simulink model "DemoCordic"  (Simulink 6.3)
settings: Solver=FixedStepDiscrete  SolverMode=SingleTasking  StartTime=0.0  StopTime=137*20*8  FixedStep=1  RelTol=1e-3
PreLoadFcn:
  | cordic_precision=20;
  | ScalingFactor = (2^(cordic_precision-1))-1;
  | K=1.0;
  | for i=1:cordic_precision
  |   cordic_atan_table(i) = round(atan(K)*ScalingFactor);
  |   K=0.5*K;
  | end;
  | disp(['cordic_precision =' num2str(cordic_precision)]);
  | disp(['cordic_atan_table =' num2str(cordic_atan_table)]);
InitFcn:
  | %% DSPBuilder Start
  | alt_dspbuilder_update_model(bdroot)
  | %% DSPBuilder End
libraries: allblocks_alteradspbuilder2 x51
settings Model: LastModifiedBy=LKONG  StrictBusMsg=None
settings DataIOCC: SignalLoggingName=sigsOut
settings OptimizationCC: InlineInvariantSignals=on
settings DebuggingCC: SolverPrmCheckMsg=none
settings HardwareCC: TargetUnknown=on

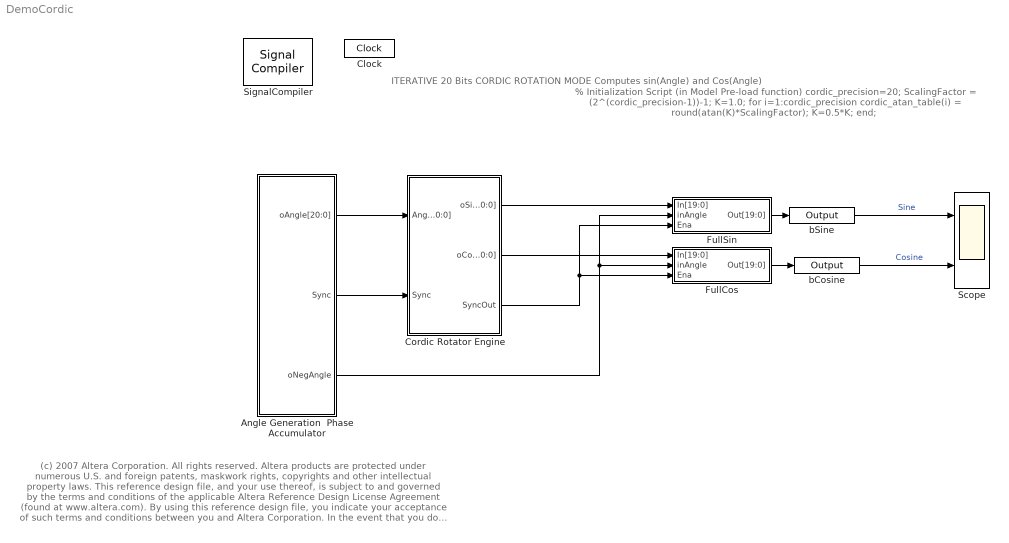
== system DemoCordic ==
  note: ITERATIVE 20 Bits CORDIC
      | ROTATION MODE
      | Computes sin(Angle) and Cos(Angle)
  note: % Initialization Script (in Model Pre-load function)
      | cordic_precision=20;
      | ScalingFactor = (2^(cordic_precision-1))-1;
      | K=1.0;
      | for i=1:cordic_precision
      |   cordic_atan_table(i) = round(atan(K)*ScalingFactor);
      |   K=0.5*K;
      | end;
  note: (c) 2007 Altera Corporation. All rights reserved.  Altera products are protected under numerous U.S. and foreign patents, maskwork rights, copyrights and other intellectual property laws.
      | This reference design file, and your use thereof, is subject to and governed by the terms and conditions of the applicable Altera Reference Design License Agreement (found at www.altera.com).
      | By using this reference design file, you indicate your acceptance of such terms and conditions between you and Altera Corporation.
      | In the event that you do not agree with such terms and conditions, you may not use the reference design file and please promptly destroy any copies you have made.
      | This reference design file being provided on an "as-is" basis and as an accommodation and therefore all warranties, representations or guarantees of any kind (whether express, implied or statutory)
      | including, without limitation, warranties of merchantability, non-infringement, or fitness for a particular purpose, are specifically disclaimed.
      | By making this reference design file available, Altera expressly does not recommend, suggest or require that this reference design file be used in combination with any other product not provided by Altera
  Angle Generation  Phase Accumulator : Subsystem  AncestorBlock=ALTELINK/AltLab/HDL SubSystem
      mask Type: SubSystem AlteraBlockSet
  Clock : allblocks_alteradspbuilder2/Clock  ClockPeriod=100  ClockPeriodUnit=ns  SampleTime=1  SimulationStartCycle=5  PhaseOffset=0  Reset=aclr  ResetType=Active Low  Export=off
  Cordic Rotator Engine : Subsystem  AncestorBlock=ALTELINK/AltLab/HDL SubSystem
      mask Type: SubSystem AlteraBlockSet
  FullCos : Subsystem  AncestorBlock=ALTELINK/AltLab/HDL SubSystem
      mask Type: SubSystem AlteraBlockSet
  FullSin : Subsystem  AncestorBlock=ALTELINK/AltLab/HDL SubSystem
      mask Type: SubSystem AlteraBlockSet
  Scope : Scope  NumInputPorts=2
      settings: YMin=-750000~-750000  YMax=750000~750000  Decimation=20
  SignalCompiler : allblocks_alteradspbuilder2/Signal Compiler  DeviceFamily=Stratix IV  DeviceName=AUTO  EnableSignalTap=off  SignalTapDepth=128  UseBoardBlock=off  StpUseDefaultClock=on  StpClock=Clock
  bCosine : allblocks_alteradspbuilder2/Output  iofile=d:\wsTrunk\workspace\Documentation\DesignExamples\Demos\Transforms\Cordic\tb_DemoCordic\DemoCordic_bCosine.capture  BusType=Signed Integer  bwl=21  bwr=0  PORTTYPE=Output
  bSine : allblocks_alteradspbuilder2/Output  iofile=d:\wsTrunk\workspace\Documentation\DesignExamples\Demos\Transforms\Cordic\tb_DemoCordic\DemoCordic_bSine.capture  BusType=Signed Integer  bwl=21  bwr=0  PORTTYPE=Output
  wires:
  bCosine/1 -> Scope/2  "Cosine"
  Cordic Rotator Engine/3(SyncOut) -> FullSin/3(Ena), FullCos/3(Ena)
  bSine/1 -> Scope/1  "Sine"
  Angle Generation  Phase Accumulator/2(Sync) -> Cordic Rotator Engine/2(Sync)
  Angle Generation  Phase Accumulator/1(oAngle[20:0]) -> Cordic Rotator Engine/1(Angle[20:0])
  Angle Generation  Phase Accumulator/3(oNegAngle) -> FullSin/2(inAngle), FullCos/2(inAngle)
  FullSin/1(Out[19:0]) -> bSine/1
  Cordic Rotator Engine/1(oSin[20:0]) -> FullSin/1(In[19:0])
  FullCos/1(Out[19:0]) -> bCosine/1
  Cordic Rotator Engine/2(oCos[20:0]) -> FullCos/1(In[19:0])

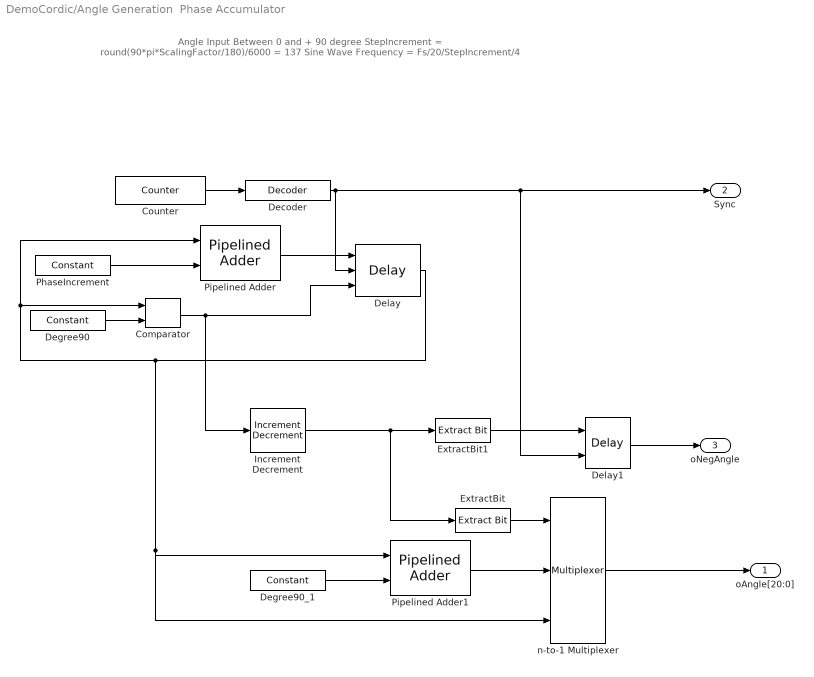
== system DemoCordic/Angle Generation  Phase Accumulator ==
  note: Angle Input Between 0 and + 90 degree
      | StepIncrement = round(90*pi*ScalingFactor/180)/6000 = 137
      | Sine Wave Frequency = Fs/20/StepIncrement/4
  Comparator : allblocks_alteradspbuilder2/Comparator  direction=a > b
  Counter : allblocks_alteradspbuilder2/Counter  BusType=Unsigned Integer  bwl=5  bwr=0  use_modulo=on  modulo=20  SpecifyClock=off  direction=Increment  use_sload=off  use_sset=off  svalue=1  use_clk_ena=off  use_ena=off  use_sclr=off
  Decoder : allblocks_alteradspbuilder2/Decoder  BusType=Unsigned Integer  bwl=5  bwr=0  registered=off  value=0
  Degree90 : allblocks_alteradspbuilder2/Constant  mask_cst=round(90*pi*ScalingFactor/180)  BusType=Signed Integer  bwl=21  bwr=0  SpecifyClock=off
  Degree90_1 : allblocks_alteradspbuilder2/Constant  mask_cst=round(90*pi*ScalingFactor/180)  BusType=Signed Integer  bwl=21  bwr=0  SpecifyClock=off
  Delay : allblocks_alteradspbuilder2/Delay  pipeline=1  ClockPhase=1  use_ena=on  use_sclr=on  use_init=off  reset_value=1
  Delay1 : allblocks_alteradspbuilder2/Delay  pipeline=2  ClockPhase=1  use_ena=on  use_sclr=off  use_init=off  reset_value=1
  ExtractBit : allblocks_alteradspbuilder2/Extract Bit  BusType=Signed Fractional  bwl=2  bwr=0  bitToSelect=0
  ExtractBit1 : allblocks_alteradspbuilder2/Extract Bit  BusType=Signed Fractional  bwl=2  bwr=0  bitToSelect=1
  Increment Decrement : allblocks_alteradspbuilder2/Increment Decrement  BusType=Unsigned Integer  bwl=2  bwr=0  SpecifyClock=off  clr_value=0  direction=Increment  phase_selection=1  use_ena=on  use_sclr=off
  PhaseIncrement : allblocks_alteradspbuilder2/Constant  mask_cst=6000  BusType=Signed Integer  bwl=21  bwr=0  SpecifyClock=off
  Pipelined Adder : allblocks_alteradspbuilder2/Pipelined Adder  BusType=Signed Integer  bwl=21  bwr=0  pipeline=0  AddSubDirection=ADD  use_cin=off  use_ovl=off  use_addsub=off  use_ena=off  use_aclr=off
  Pipelined Adder1 : allblocks_alteradspbuilder2/Pipelined Adder  BusType=Signed Integer  bwl=21  bwr=0  pipeline=0  AddSubDirection=SUB  use_cin=off  use_ovl=off  use_addsub=off  use_ena=off  use_aclr=off
  n-to-1 Multiplexer : allblocks_alteradspbuilder2/Multiplexer  numInputs=2  pipeline=0  oneHot=off  use_ena=off  use_aclr=off
  oAngle[20:0] : Outport
  Sync : Outport  Port=2
  oNegAngle : Outport  Port=3
  wires:
  Counter/1 -> Decoder/1
  Decoder/1 -> Delay/2, Delay1/2, Sync/1
  Pipelined Adder/1 -> Delay/1
  PhaseIncrement/1 -> Pipelined Adder/2
  Delay/1 -> Comparator/1, Pipelined Adder/1, n-to-1 Multiplexer/3, Pipelined Adder1/1
  Comparator/1 -> Delay/3, Increment Decrement/1
  Degree90/1 -> Comparator/2
  Increment Decrement/1 -> ExtractBit/1, ExtractBit1/1
  n-to-1 Multiplexer/1 -> oAngle[20:0]/1
  Pipelined Adder1/1 -> n-to-1 Multiplexer/2
  Degree90_1/1 -> Pipelined Adder1/2
  ExtractBit/1 -> n-to-1 Multiplexer/1
  Delay1/1 -> oNegAngle/1
  ExtractBit1/1 -> Delay1/1

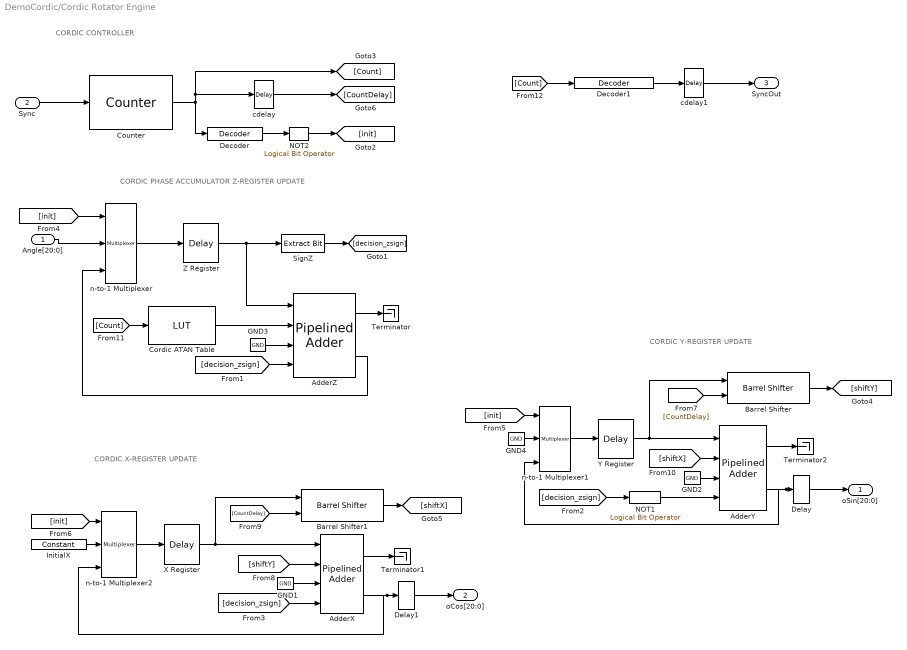
== system DemoCordic/Cordic Rotator Engine ==
  note: CORDIC CONTROLLER
  note: CORDIC PHASE ACCUMULATOR Z-REGISTER UPDATE
  note: CORDIC X-REGISTER UPDATE
  note: CORDIC Y-REGISTER UPDATE
  Angle[20:0] : Inport
  Sync : Inport  Port=2
  AdderX : allblocks_alteradspbuilder2/Pipelined Adder  BusType=Signed Integer  bwl=21  bwr=0  pipeline=0  AddSubDirection=ADD  use_cin=on  use_ovl=on  use_addsub=on  use_ena=on  use_aclr=on
  AdderY : allblocks_alteradspbuilder2/Pipelined Adder  BusType=Signed Integer  bwl=21  bwr=0  pipeline=0  AddSubDirection=ADD  use_cin=on  use_ovl=on  use_addsub=on  use_ena=on  use_aclr=on
  AdderZ : allblocks_alteradspbuilder2/Pipelined Adder  BusType=Signed Integer  bwl=21  bwr=0  pipeline=0  AddSubDirection=ADD  use_cin=on  use_ovl=on  use_addsub=on  use_ena=on  use_aclr=on
  Barrel Shifter : allblocks_alteradspbuilder2/Barrel Shifter  BusType=Signed Integer  bwl=20  bwr=0  pipeline=off  ShiftDirection=Shift right  use_ena=off  use_aclr=off  UseDedicatedCircuitry=off
  Barrel Shifter1 : allblocks_alteradspbuilder2/Barrel Shifter  BusType=Signed Integer  bwl=20  bwr=0  pipeline=off  ShiftDirection=Shift right  use_ena=off  use_aclr=off  UseDedicatedCircuitry=off
  "Cordic ATAN Table " : allblocks_alteradspbuilder2/LUT  addr_width=5  BusType=Signed Integer  bwl=20  bwr=0  init_array=cordic_atan_table  use_ena=off  reg_data=off  use_lpm=off  reg_addr=on  ram_type=AUTO
  Counter : allblocks_alteradspbuilder2/Counter  BusType=Unsigned Integer  bwl=5  bwr=0  use_modulo=on  modulo=20  SpecifyClock=off  direction=Increment  use_sload=off  use_sset=off  svalue=1  use_clk_ena=off  use_ena=off  use_sclr=on
  Decoder : allblocks_alteradspbuilder2/Decoder  BusType=Unsigned Integer  bwl=5  bwr=0  registered=off  value=0
  Decoder1 : allblocks_alteradspbuilder2/Decoder  BusType=Unsigned Integer  bwl=5  bwr=0  registered=off  value=19
  Delay : allblocks_alteradspbuilder2/Delay  pipeline=1  ClockPhase=1  use_ena=off  use_sclr=off  use_init=off  reset_value=1
  Delay1 : allblocks_alteradspbuilder2/Delay  pipeline=1  ClockPhase=1  use_ena=off  use_sclr=off  use_init=off  reset_value=1
  GND{1..4} (4 alike) : allblocks_alteradspbuilder2/GND  SpecifyClock=off
  InitialX : allblocks_alteradspbuilder2/Constant  mask_cst=round(0.60725293510314*ScalingFactor)  BusType=Signed Integer  bwl=20  bwr=0  SpecifyClock=off
  NOT1 : allblocks_alteradspbuilder2/Logical Bit Operator  LogicalOperator=NOT  user_inputs=2
  NOT2 : allblocks_alteradspbuilder2/Logical Bit Operator  LogicalOperator=NOT  user_inputs=2
  SignZ : allblocks_alteradspbuilder2/Extract Bit  BusType=Signed Fractional  bwl=21  bwr=0  bitToSelect=20
  Terminator : Terminator
  Terminator1 : Terminator
  Terminator2 : Terminator
  X Register : allblocks_alteradspbuilder2/Delay  pipeline=1  ClockPhase=1  use_ena=off  use_sclr=off  use_init=off  reset_value=1
  Y Register : allblocks_alteradspbuilder2/Delay  pipeline=1  ClockPhase=1  use_ena=off  use_sclr=off  use_init=off  reset_value=1
  Z Register : allblocks_alteradspbuilder2/Delay  pipeline=1  ClockPhase=1  use_ena=off  use_sclr=off  use_init=off  reset_value=1
  cdelay : allblocks_alteradspbuilder2/Delay  pipeline=1  ClockPhase=1  use_ena=off  use_sclr=off  use_init=off  reset_value=1
  cdelay1 : allblocks_alteradspbuilder2/Delay  pipeline=2  ClockPhase=1  use_ena=off  use_sclr=off  use_init=off  reset_value=1
  n-to-1 Multiplexer : allblocks_alteradspbuilder2/Multiplexer  numInputs=2  pipeline=0  oneHot=off  use_ena=off  use_aclr=off
  n-to-1 Multiplexer1 : allblocks_alteradspbuilder2/Multiplexer  numInputs=2  pipeline=0  oneHot=off  use_ena=off  use_aclr=off
  n-to-1 Multiplexer2 : allblocks_alteradspbuilder2/Multiplexer  numInputs=2  pipeline=0  oneHot=off  use_ena=off  use_aclr=off
  oSin[20:0] : Outport
  oCos[20:0] : Outport  Port=2
  SyncOut : Outport  Port=3
  wires:
  Angle[20:0]/1 -> n-to-1 Multiplexer/2
  Sync/1 -> Counter/1
  GND1/1 -> AdderX/3
  GND2/1 -> AdderY/3
  AdderX/2 -> n-to-1 Multiplexer2/3, Delay1/1
  AdderY/2 -> n-to-1 Multiplexer1/3, Delay/1
  Y Register/1 -> AdderY/1, Barrel Shifter/1
  X Register/1 -> AdderX/1, Barrel Shifter1/1
  n-to-1 Multiplexer/1 -> Z Register/1
  GND3/1 -> AdderZ/3
  Z Register/1 -> AdderZ/1, SignZ/1
  SignZ/1 -> [decision_zsign]
  [decision_zsign] -> AdderZ/4
  NOT1/1 -> AdderY/4
  [decision_zsign] -> NOT1/1
  Decoder/1 -> NOT2/1
  [init] -> n-to-1 Multiplexer/1
  [init] -> n-to-1 Multiplexer1/1
  n-to-1 Multiplexer1/1 -> Y Register/1
  GND4/1 -> n-to-1 Multiplexer1/2
  [decision_zsign] -> AdderX/4
  [init] -> n-to-1 Multiplexer2/1
  InitialX/1 -> n-to-1 Multiplexer2/2
  n-to-1 Multiplexer2/1 -> X Register/1
  [CountDelay] -> Barrel Shifter/2
  Barrel Shifter/1 -> [shiftY]
  [shiftY] -> AdderX/2
  [CountDelay] -> Barrel Shifter1/2
  Barrel Shifter1/1 -> [shiftX]
  [shiftX] -> AdderY/2
  "Cordic ATAN Table "/1 -> AdderZ/2
  [Count] -> "Cordic ATAN Table "/1
  Counter/1 -> Decoder/1, cdelay/1, [Count]
  AdderZ/2 -> n-to-1 Multiplexer/3
  NOT2/1 -> [init]
  cdelay/1 -> [CountDelay]
  Decoder1/1 -> cdelay1/1
  cdelay1/1 -> SyncOut/1
  [Count] -> Decoder1/1
  Delay1/1 -> oCos[20:0]/1
  AdderZ/1 -> Terminator/1
  AdderX/1 -> Terminator1/1
  AdderY/1 -> Terminator2/1
  Delay/1 -> oSin[20:0]/1

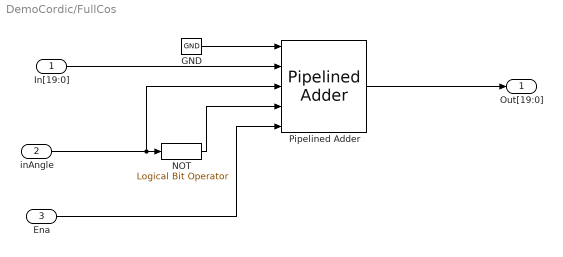
== system DemoCordic/FullCos ==
  In[19:0] : Inport
  inAngle : Inport  Port=2
  Ena : Inport  Port=3
  GND : allblocks_alteradspbuilder2/GND  SpecifyClock=off
  NOT : allblocks_alteradspbuilder2/Logical Bit Operator  LogicalOperator=NOT  user_inputs=2
  Pipelined Adder : allblocks_alteradspbuilder2/Pipelined Adder  BusType=Signed Integer  bwl=20  bwr=0  pipeline=2  AddSubDirection=ADD  use_cin=on  use_ovl=off  use_addsub=on  use_ena=on  use_aclr=off
  Out[19:0] : Outport
  wires:
  Ena/1 -> Pipelined Adder/5
  GND/1 -> Pipelined Adder/1
  NOT/1 -> Pipelined Adder/4
  In[19:0]/1 -> Pipelined Adder/2
  inAngle/1 -> Pipelined Adder/3, NOT/1
  Pipelined Adder/1 -> Out[19:0]/1

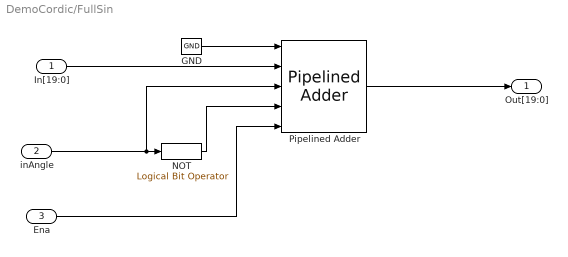
== system DemoCordic/FullSin ==
  In[19:0] : Inport
  inAngle : Inport  Port=2
  Ena : Inport  Port=3
  GND : allblocks_alteradspbuilder2/GND  SpecifyClock=off
  NOT : allblocks_alteradspbuilder2/Logical Bit Operator  LogicalOperator=NOT  user_inputs=2
  Pipelined Adder : allblocks_alteradspbuilder2/Pipelined Adder  BusType=Signed Integer  bwl=20  bwr=0  pipeline=2  AddSubDirection=ADD  use_cin=on  use_ovl=off  use_addsub=on  use_ena=on  use_aclr=off
  Out[19:0] : Outport
  wires:
  inAngle/1 -> NOT/1, Pipelined Adder/3
  In[19:0]/1 -> Pipelined Adder/2
  NOT/1 -> Pipelined Adder/4
  GND/1 -> Pipelined Adder/1
  Pipelined Adder/1 -> Out[19:0]/1
  Ena/1 -> Pipelined Adder/5
